simulink model "cascade_time"  (R2019b)
settings: Solver=VariableStepAuto  StartTime=0.0  StopTime=10.0  RelTol=1e-3
settings Model: Creator=davis  LastModifiedBy=davis

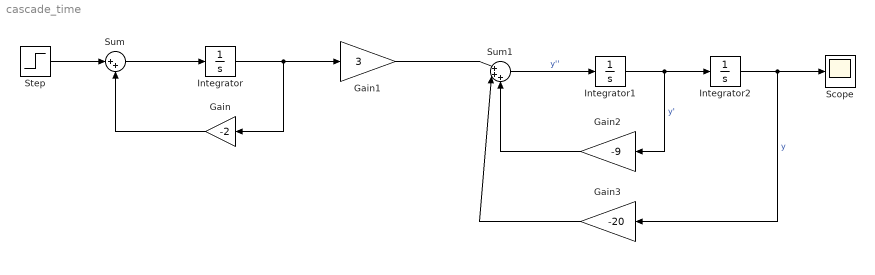
== system cascade_time ==
  Gain : Gain  Gain=-2
  Gain1 : Gain  Gain=3
  Gain2 : Gain  Gain=-9
  Gain3 : Gain  Gain=-20
  Integrator : Integrator  InitialCondition=1
  Integrator1 : Integrator  InitialCondition=2
  Integrator2 : Integrator  InitialCondition=3
  Scope : Scope
  Step : Step  Time=0  SampleTime=0
  Sum : Sum  Inputs=|++
  Sum1 : Sum  Inputs=|+++
  wires:
  Sum/1 -> Integrator/1
  Integrator/1 -> Gain1/1, Gain/1
  Step/1 -> Sum/1
  Gain/1 -> Sum/2
  Gain2/1 -> Sum1/3
  Integrator1/1 -> Gain2/1, Integrator2/1  "y'"
  Sum1/1 -> Integrator1/1  "y''"
  Gain1/1 -> Sum1/1
  Gain3/1 -> Sum1/2
  Integrator2/1 -> Gain3/1, Scope/1  "y"
